simulink library "INT_Tra_DblClthDet"  (R2016b)
settings: Solver=VariableStepAuto  StartTime=0.0  StopTime=10.0  RelTol=1e-3
settings Model: Creator=Administrator  LastModifiedBy=Administrator

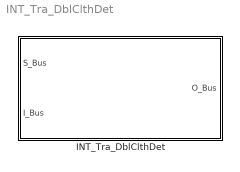
== system INT_Tra_DblClthDet ==
  INT_Tra_DblClthDet : Subsystem

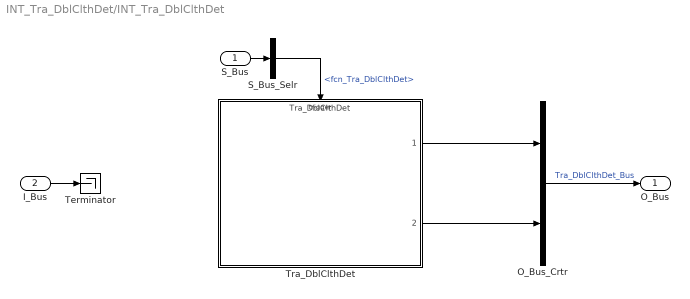
== system INT_Tra_DblClthDet/INT_Tra_DblClthDet ==
  S_Bus : Inport
  I_Bus : Inport  Port=2
  O_Bus_Crtr : BusCreator  Inputs=2
  S_Bus_Selr : BusSelector  OutputSignals=fcn_Tra_DblClthDet
  Terminator : Terminator
  Tra_DblClthDet : ModelReference  ModelNameDialog=Tra_DblClthDet  SimulationMode=Normal  ModelReferenceVersion=1.5  TriggerPortName=function  TriggerPortTriggerType=function-call  TriggerPortStatesWhenEnabling=held
  O_Bus : Outport
  wires:
  S_Bus_Selr/1 -> Tra_DblClthDet/Trigger  "<fcn_Tra_DblClthDet>"
  S_Bus/1 -> S_Bus_Selr/1
  I_Bus/1 -> Terminator/1
  O_Bus_Crtr/1 -> O_Bus/1  "Tra_DblClthDet_Bus"
  Tra_DblClthDet/1 -> O_Bus_Crtr/1
  Tra_DblClthDet/2 -> O_Bus_Crtr/2
